simulink model "model_02"  (R2021b)
settings: Solver=ode45  StartTime=0.0  StopTime=10  RelTol=1e-3
settings Model: Creator=jimd  LastModifiedBy=jim

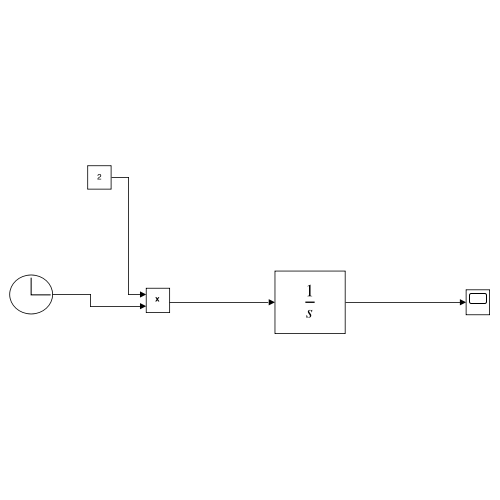
[thumbnail: Simulink's stored preview of the top-level diagram]
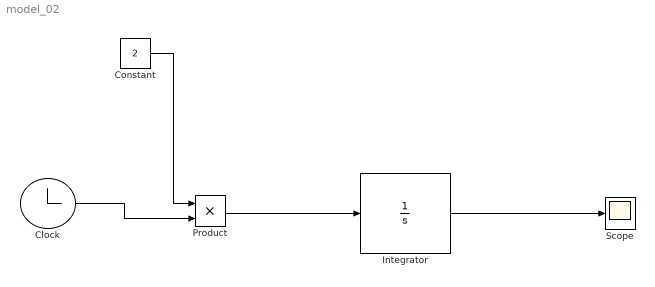
== system model_02 ==
  Clock : Clock
  Constant : Constant  Value=2
  Integrator : Integrator
  Product : Product
  Scope : Scope
  wires:
  Constant/1 -> Product/1
  Clock/1 -> Product/2
  Product/1 -> Integrator/1
  Integrator/1 -> Scope/1
